simulink model "CD_CD_simulink"  (R2023b)
settings: Solver=VariableStepAuto  StartTime=0.0  StopTime=0.01  RelTol=1e-3
settings Model: Creator=penqu  LastModifiedBy=penqu

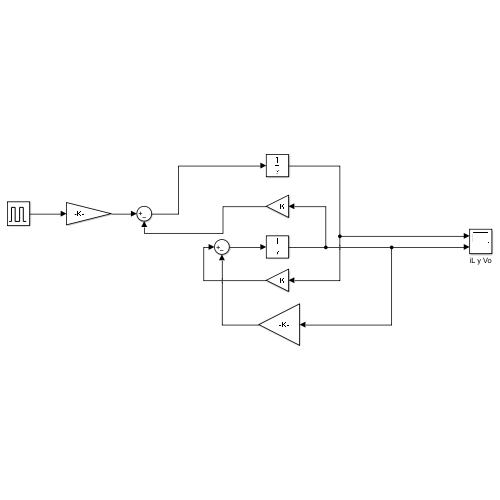
[thumbnail: Simulink's stored preview of the top-level diagram]
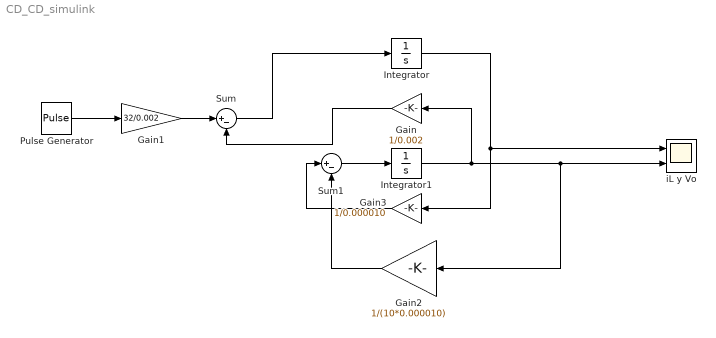
== system CD_CD_simulink ==
  Gain : Gain  Gain=1/0.002
  Gain1 : Gain  Gain=32/0.002
  Gain2 : Gain  Gain=1/(10*0.000010)
  Gain3 : Gain  Gain=1/0.000010
  Integrator : Integrator
  Integrator1 : Integrator
  Pulse Generator : DiscretePulseGenerator  PulseType=Time based  Amplitude=0.955  Period=1e-5  PulseWidth=40
  Sum : Sum  Inputs=|+-
  Sum1 : Sum  Inputs=|+-
  iL y Vo : Scope  NumInputPorts=2
  wires:
  Integrator/1 -> Gain3/1, iL y Vo/1
  Gain2/1 -> Sum1/2
  Gain/1 -> Sum/2
  Gain3/1 -> Sum1/1
  Sum1/1 -> Integrator1/1
  Pulse Generator/1 -> Gain1/1
  Sum/1 -> Integrator/1
  Integrator1/1 -> Gain/1, Gain2/1, iL y Vo/2
  Gain1/1 -> Sum/1
